simulink model "SMCFinalSim"  (R2024a)
settings: Solver=VariableStepAuto  StartTime=0.0  StopTime=80  RelTol=1e-3
undefined symbols (not defined in the file): a, Aa, Bb, beta, betaF, C, g, J, Kf, l, Lb, Lm, m_b, m_m
settings Model: Creator=Cami  LastModifiedBy=alfar

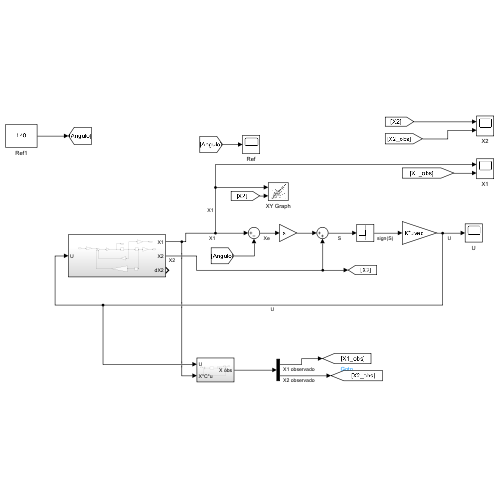
[thumbnail: Simulink's stored preview of the top-level diagram]
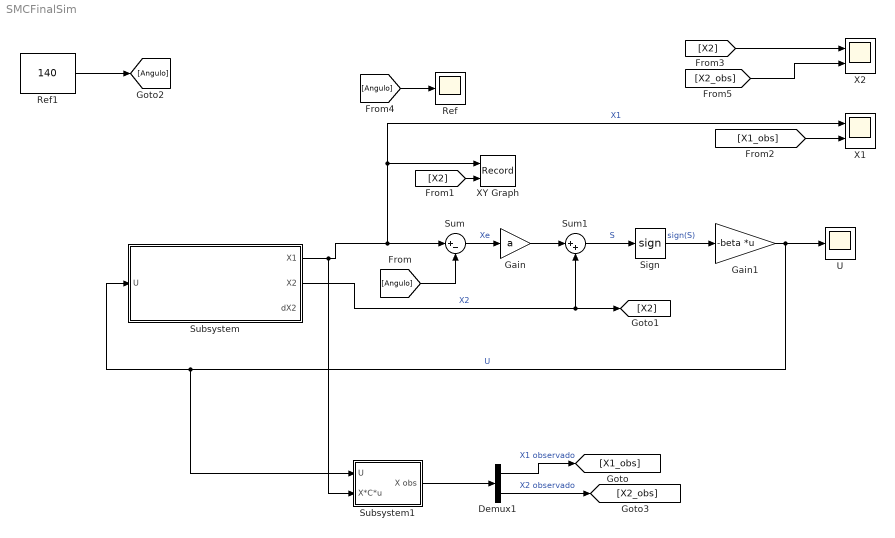
== system SMCFinalSim ==
  Demux1 : Demux  Outputs=2
  Gain : Gain  Gain=a
  Gain1 : Gain  Gain=-beta  Multiplication=Matrix(K*u) (u vector)
  Ref : Scope
  Ref1 : Constant  Value=140
  Sign : Signum  ZeroCross=off
  Subsystem : Subsystem
  Subsystem1 : Subsystem
  Sum : Sum  Inputs=|+-
  Sum1 : Sum  Inputs=|++
  U : Scope
  X1 : Scope  NumInputPorts=2
  X2 : Scope  NumInputPorts=2
  XY Graph : Record  FileSettingsInternal="{\"entries\":[{\"content\":{\"excelSettings\":{\"content\":{},\"type\":\"Streamout.ExcelSettings\"}},\"type\":\"Streamout.FileSettingStorage\",\"uuid\":\"\"}],\"packageUris\":[\"http:\\/\\/schema.mathworks.com\\/mf0\\/streamout_blocks\\/R2020a\"],\"version\":\"1.0\"}"  Layout=[1 1]  SignalsInternal="{\"entries\":[{\"content\":{\"signals\":[{\"content\":{\"blockPath\":[],\"dimensions\":[1],\"domain\":\"\",\"lineColor\":\"#a2142f\",\"plots\":[ 1 ],\"port\":1,\"sid\":[\"\"],\"signalID\":1,\"signalName\":\"X1\"},\"type\":\"RecordBlkView.Signal\",\"uuid\":\"\"},{\"content\":{\"blockPath\":[],\"dimensions\":[1],\"domain\":\"\",\"lineColor\":\"#139fff\",\"plots\":[ 1 ],\"port\":2,\"sid\":[\"\"],\"signalID\":2,\"signalName\":\"From1\"},\"type\":\"RecordBlkView.Signal\",\"uuid\":\"\"}]},\"type\":\"RecordBlkView.InputSignals\",\"uuid\":\"\"}],\"packageUris\":[\"http:\\/\\/schema.mathworks.com\\/mf0\\/streamout_blocks\\/R2020a\"],\"version\":\"1.0\"}"  VisualizationBindings="{\"xyplotplugin\":{\"info\":[{\"series\":[{\"bindingParametersList\":[{\"parameter\":\"X-Axis\",\"signalID\":1,\"signalName\":\"X1\"},{\"parameter\":\"Y-Axis\",\"signalID\":2,\"signalName\":\"From1\"}],\"seriesID\":0}],\"subplotID\":1}]}}"  CompatibilityTag=XY
  wires:
  Sum/1 -> Gain/1  "Xe"
  Gain1/1 -> Subsystem1/1(U), Subsystem/1(U), U/1  "U"
  [X2] -> X2/1
  Sign/1 -> Gain1/1  "sign(S)"
  Sum1/1 -> Sign/1  "S"
  Gain/1 -> Sum1/1
  [X2] -> XY Graph/2
  Subsystem/1(X1) -> Subsystem1/2(X*C*u), Sum/1, X1/1, XY Graph/1  "X1"
  [Angulo] -> Sum/2
  Ref1/1 -> [Angulo]
  Subsystem1/1(X obs) -> Demux1/1
  [Angulo] -> Ref/1
  Subsystem/2(X2) -> Sum1/2, [X2]  "X2"
  Demux1/1 -> [X1_obs]  "X1 observado"
  [X1_obs] -> X1/2
  Demux1/2 -> [X2_obs]  "X2 observado"
  [X2_obs] -> X2/2

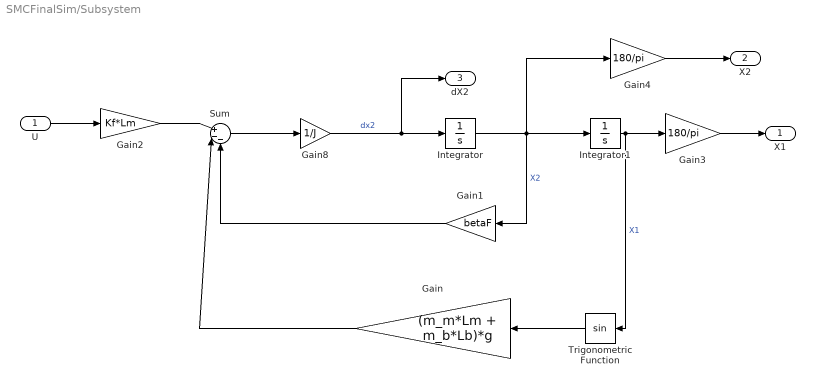
== system SMCFinalSim/Subsystem ==
  U : Inport
  Gain : Gain  Gain=(m_m*Lm + m_b*Lb)*g
  Gain1 : Gain  Gain=betaF
  Gain2 : Gain  Gain=Kf*Lm
  Gain3 : Gain  Gain=180/pi
  Gain4 : Gain  Gain=180/pi
  Gain8 : Gain  Gain=1/J
  Integrator : Integrator
  Integrator1 : Integrator
  Sum : Sum  Inputs=|+--
  Trigonometric Function : Trigonometry
  X1 : Outport
  X2 : Outport  Port=2
  dX2 : Outport  Port=3
  wires:
  U/1 -> Gain2/1
  Gain1/1 -> Sum/3
  Gain/1 -> Sum/2
  Gain2/1 -> Sum/1
  Integrator1/1 -> Gain3/1, Trigonometric Function/1  "X1"
  Trigonometric Function/1 -> Gain/1
  Sum/1 -> Gain8/1
  Integrator/1 -> Gain4/1, Gain1/1, Integrator1/1  "X2"
  Gain8/1 -> dX2/1, Integrator/1  "dx2"
  Gain3/1 -> X1/1
  Gain4/1 -> X2/1

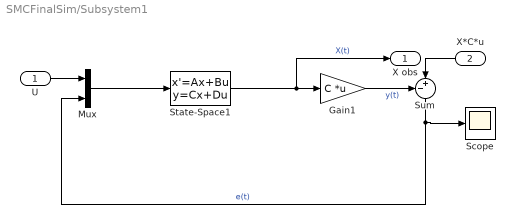
== system SMCFinalSim/Subsystem1 ==
  U : Inport
  X*C*u : Inport  Port=2
  Gain1 : Gain  Gain=C  Multiplication=Matrix(K*u)
  Mux : Mux  Inputs=2
  Scope : Scope
  State-Space1 : StateSpace  A=Aa  B=[Bb l']  C=eye(2)  D=zeros(2,2)  InitialCondition=0
  Sum : Sum  Inputs=-+|
  X obs : Outport
  wires:
  Sum/1 -> Scope/1, Mux/2  "e(t)"
  Gain1/1 -> Sum/1  "y(t)"
  Mux/1 -> State-Space1/1
  U/1 -> Mux/1
  State-Space1/1 -> X obs/1, Gain1/1  "X(t)"
  X*C*u/1 -> Sum/2
